simulink model "dsplpc_win32"  (Simulink 6.0)
settings: Solver=FixedStepDiscrete  SolverMode=SingleTasking  StartTime=0.0  StopTime=0.49  RelTol=1e-3
PreLoadFcn:
  | load mtlb;
libraries: dsparch4 x4, dspsrcs4 x1, dspstat3 x1, dspsolvers x1, dspbuff3 x1, dspsigops x1, dspwin32 x1
settings Model: RequirementInfo=9  Creator=dshpak  LastModifiedBy=mlongfri  ExtModeTrigMode=oneshot  ExtModeArmWhenConnect=off  ProdHWDeviceType=Specified
settings DataIOCC: LimitDataPoints=off  SaveOutput=off  SaveTime=off  SignalLoggingName=sigsOut
settings OptimizationCC: BlockReduction=off  BooleanDataType=off  InlineInvariantSignals=off  MultiInstanced=off
settings FormatCC: IgnoreBidirectionalLines=off
settings DebuggingCC: SingleTaskRateTransMsg=error  IntegerOverflowMsg=none
settings HardwareCC: ProdHWDeviceType=Specified
settings CodeAppCC: SimulinkBlockComments=off
settings GRTTargetCC: TargetFcnLib=iso_c_tmw.mat

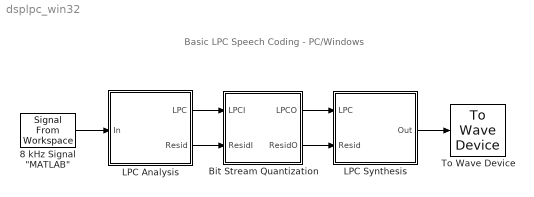
== system dsplpc_win32 ==
  note: Basic LPC Speech Coding - PC/Windows
  "8 kHz Signal \"MATLAB\"" : dspsrcs4/Signal From Workspace  X=mtlb  Ts=1/8000  nsamps=80  OutputAfterFinalValue=Setting to zero
  Bit Stream Quantization : Subsystem
  LPC Analysis : Subsystem
  LPC Synthesis : Subsystem
  To Wave Device : dspwin32/To Wave Device  bufDuration=1  initDelay=0.0  useDefaultDevice=on  enable24Bit=off
  wires:
  LPC Analysis/1(LPC) -> Bit Stream Quantization/1(LPCI)
  LPC Analysis/2(Resid) -> Bit Stream Quantization/2(ResidI)
  "8 kHz Signal \"MATLAB\""/1 -> LPC Analysis/1(In)
  Bit Stream Quantization/2(ResidO) -> LPC Synthesis/2(Resid)
  Bit Stream Quantization/1(LPCO) -> LPC Synthesis/1(LPC)
  LPC Synthesis/1(Out) -> To Wave Device/1

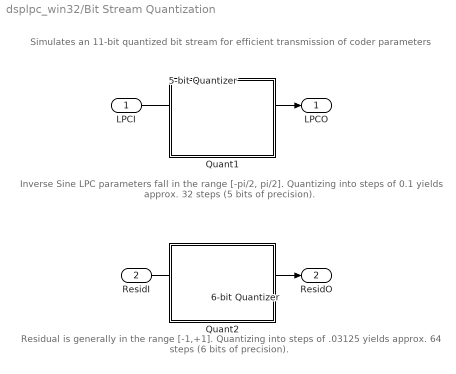
== system dsplpc_win32/Bit Stream Quantization ==
  note: Inverse Sine LPC parameters fall in
      | the range [-pi/2, pi/2].  Quantizing
      | into steps of 0.1 yields approx. 32 steps
      | (5 bits of precision).
  note: Residual is generally in the range [-1,+1].
      | Quantizing into steps of .03125 yields
      | approx. 64 steps (6 bits of precision).
  note: Simulates an 11-bit quantized bit stream
      | for efficient transmission of coder parameters
  LPCI : Inport
  ResidI : Inport  Port=2
  5-bit Quantizer : Quantizer  QuantizationInterval=0.1  LinearizeAsGain=off
  6-bit Quantizer : Quantizer  QuantizationInterval=0.03125  LinearizeAsGain=off
  Quant1 : Subsystem
      mask Display: disp('')
  Quant2 : Subsystem
      mask Display: disp('')
  LPCO : Outport
  ResidO : Outport  Port=2
  wires:
  6-bit Quantizer/1 -> ResidO/1
  ResidI/1 -> 6-bit Quantizer/1
  5-bit Quantizer/1 -> LPCO/1
  LPCI/1 -> 5-bit Quantizer/1

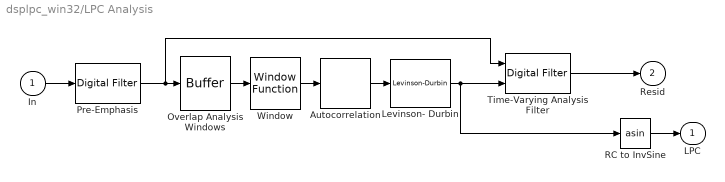
== system dsplpc_win32/LPC Analysis ==
  In : Inport
  Autocorrelation : dspstat3/Autocorrelation  DialogController=dspDDGCreate  DialogControllerArgs=DataTag0  AllPositiveLags=off  maxlag=10  bias=Biased  domain=Time  roundingMode=Floor  overflowMode=off
  Levinson- Durbin : dspsolvers/Levinson-Durbin  DialogController=dspDDGCreate  DialogControllerArgs=DataTag1  coeffOutFcn=K  outP=off  zeroInpHandling=on  firstCoeffMode=Binary point scaling  firstCoeffWordLength=16  firstCoeffFracLength=15  secondCoeffMode=Binary point scaling  secondCoeffWordLength=16  secondCoeffFracLength=15  roundingMode=Floor  overflowMode=off
      settings: allowOverrides=off
  Overlap Analysis Windows : dspbuff3/Buffer  N=160  V=80  ic=0
  Pre-Emphasis : dsparch4/Digital Filter  TypePopup=FIR (all zeros)  IIRFiltStruct=Direct form II transposed  AllPoleFiltStruct=Direct form  FIRFiltStruct=Direct form  CoeffSource=Specify via dialog  NumCoeffs=[1 -.95] / 3.0  DenCoeffs=[1 0.1]  BiQuadCoeffs=[1 0.3 0.4 1 0.1 0.2]  LatticeCoeffs=[0.2 0.4]  denIgnore=on  FiltPerSampPopup=One filter per frame  IC=0  ICnum=0  ICden=0  roundingMode=Floor  overflowMode=off
  RC to InvSine : Trigonometry  Operator=asin
  Time-Varying Analysis Filter : dsparch4/Digital Filter  TypePopup=FIR (all zeros)  IIRFiltStruct=Direct form II transposed  AllPoleFiltStruct=Direct form  FIRFiltStruct=Lattice MA  CoeffSource=Input port(s)  NumCoeffs=[1 -.95] / 3.0  DenCoeffs=[1 0.1]  BiQuadCoeffs=[1 0.3 0.4 1 0.1 0.2]  LatticeCoeffs=[0.2 0.4]  denIgnore=on  FiltPerSampPopup=One filter per frame  IC=0  ICnum=0  ICden=0  roundingMode=Floor  overflowMode=off
  Window : dspsigops/Window Function  winmode=Apply window to input  wintype=Hamming  sampmode=Continuous  samptime=1  N=64  Rs=50  beta=10  winsamp=Symmetric  UserWindow=hamming  OptParams=off  UserParams={1.0}  dataType=double  isSigned=on  wordLen=16  udDataType=sfix(16)  fracBitsMode=Best precision  numFracBits=15  roundingMode=Floor  overflowMode=off
  LPC : Outport
  Resid : Outport  Port=2
  wires:
  Pre-Emphasis/1 -> Overlap Analysis Windows/1, Time-Varying Analysis Filter/1
  Overlap Analysis Windows/1 -> Window/1
  Autocorrelation/1 -> Levinson- Durbin/1
  Window/1 -> Autocorrelation/1
  Levinson- Durbin/1 -> RC to InvSine/1, Time-Varying Analysis Filter/2
  RC to InvSine/1 -> LPC/1
  In/1 -> Pre-Emphasis/1
  Time-Varying Analysis Filter/1 -> Resid/1

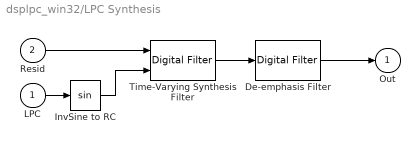
== system dsplpc_win32/LPC Synthesis ==
  LPC : Inport
  Resid : Inport  Port=2
  De-emphasis Filter : dsparch4/Digital Filter  TypePopup=IIR (all poles)  IIRFiltStruct=Direct form II transposed  AllPoleFiltStruct=Direct form  FIRFiltStruct=Direct form  CoeffSource=Specify via dialog  NumCoeffs=[1 -.95] / 3.0  DenCoeffs=[1 -.95]  BiQuadCoeffs=[1 0.3 0.4 1 0.1 0.2]  LatticeCoeffs=[0.2 0.4]  denIgnore=on  FiltPerSampPopup=One filter per frame  IC=0  ICnum=0  ICden=0  roundingMode=Floor  overflowMode=off
  InvSine to RC : Trigonometry
  Time-Varying Synthesis Filter : dsparch4/Digital Filter  TypePopup=IIR (all poles)  IIRFiltStruct=Direct form II transposed  AllPoleFiltStruct=Lattice AR  FIRFiltStruct=Direct form  CoeffSource=Input port(s)  NumCoeffs=[1 -.95] / 3.0  DenCoeffs=[1 0.1]  BiQuadCoeffs=[1 0.3 0.4 1 0.1 0.2]  LatticeCoeffs=[0.2 0.4]  denIgnore=on  FiltPerSampPopup=One filter per frame  IC=0  ICnum=0  ICden=0  roundingMode=Floor  overflowMode=off
  Out : Outport
  wires:
  Time-Varying Synthesis Filter/1 -> De-emphasis Filter/1
  Resid/1 -> Time-Varying Synthesis Filter/1
  LPC/1 -> InvSine to RC/1
  InvSine to RC/1 -> Time-Varying Synthesis Filter/2
  De-emphasis Filter/1 -> Out/1

== system dsplpc_win32/Bit Stream Quantization/Quant1 ==

== system dsplpc_win32/Bit Stream Quantization/Quant2 ==
